simulink model "EMB_LRM"  (R2025a)
settings: Solver=VariableStepAuto  StartTime=0.0  StopTime=10.0  RelTol=1e-3
values from neighbouring files (symbols this model uses):
  cal_u16FailWatchWindow = uint16(20)    [sim_test.m]
  cal_u16FallbackSupportSwapTime = uint16(50)    [sim_test.m]
  cal_u16LaneInitWaitTime = uint16(100)    [sim_test.m]
  cal_u16MasterFallbackSwapThd = uint16(20)    [sim_test.m]
  cal_u16TakeoverTime = uint16(50)    [sim_test.m]
  cal_u8RmtLaneFailThd = uint8(20)    [sim_test.m]
  cal_u8RoleChangeDebounceTime = uint8(10)    [sim_test.m]
settings Model: Creator=wangtianqi  LastModifiedBy=wangtianqi

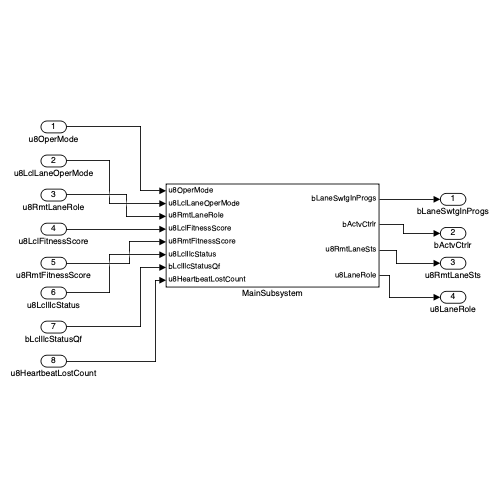
[thumbnail: Simulink's stored preview of the top-level diagram]
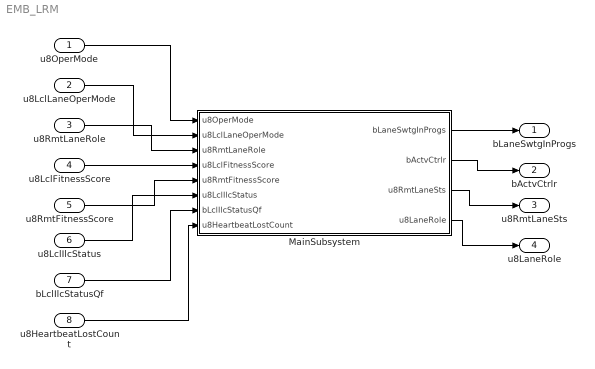
== system EMB_LRM ==
  u8OperMode : Inport  Description=系统运行模式（enum：0 INIT，1 NORMAL_OPERATION，2 LIMP_HOME，3 LIMP_ASIDE，4 CRAWL，5 SHUTTING_DOWN），类型 uint8  OutDataTypeStr=uint8
  u8LclLaneOperMode : Inport  Description=本控制链路运行模式（enum，编码同 OPER MODE），类型 uint8  Port=2  OutDataTypeStr=uint8
  u8RmtLaneRole : Inport  Description=远控制链路当前角色（enum：0 INIT，1 MASTER，2 FALLBACK，3 SUPPORT，4 DISABLED，5 SHUTTING_DOWN），类型 uint8  Port=3  OutDataTypeStr=uint8
  u8LclFitnessScore : Inport  Description=本控制链路健康度得分（62=禁用，255=无效），类型 uint8  Port=4  OutDataTypeStr=uint8
  u8RmtFitnessScore : Inport  Description=远控制链路健康度得分（62=禁用，255=无效），类型 uint8  Port=5  OutDataTypeStr=uint8
  u8LclIlcStatus : Inport  Description=本控制链路 ILC 状态（0x0 Failed，0x1 Normal，0x2 Initialized），类型 uint8  Port=6  OutDataTypeStr=uint8
  bLclIlcStatusQf : Inport  Description=本控制链路状态信号质量（0x0 QF_Full，0x1 QF_Not Full），类型 boolean  Port=7  OutDataTypeStr=boolean
  u8HeartbeatLostCount : Inport  Description=心跳丢失计数（0-255），类型 uint8  Port=8  OutDataTypeStr=uint8
  MainSubsystem : Subsystem  Description=EMB_LRM 主逻辑包装层：SignalAcquisition -> 功能子系统(LRM_MLS / LRM_MLR -> LRM_LSP) -> OutputArbitration -> Out；运行周期 10ms，ASIL-D
  bLaneSwtgInProgs : Outport  Description=控制链路切换进行中标志（0x0 Not Progress，0x1 Progress），类型 boolean  OutDataTypeStr=boolean
  bActvCtrlr : Outport  Description=活动控制器实例标志（0x0 Not Active，0x1 Active），类型 boolean  Port=2  OutDataTypeStr=boolean
  u8RmtLaneSts : Outport  Description=远控制链路状态（0 INITIALISING，1 OPERATING，2 HB_LOST，3 FAILED），类型 uint8  Port=3  OutDataTypeStr=uint8
  u8LaneRole : Outport  Description=本控制链路角色状态（enum：0 UNKNOWN，1 INIT，2 MASTER，3 FALLBACK，4 SUPPORT，5 DISABLED，6 SHUTTING_DOWN），类型 uint8  Port=4  OutDataTypeStr=uint8
  wires:
  MainSubsystem/4(u8LaneRole) -> u8LaneRole/1
  u8RmtLaneRole/1 -> MainSubsystem/3(u8RmtLaneRole)
  u8OperMode/1 -> MainSubsystem/1(u8OperMode)
  MainSubsystem/2(bActvCtrlr) -> bActvCtrlr/1
  MainSubsystem/1(bLaneSwtgInProgs) -> bLaneSwtgInProgs/1
  u8HeartbeatLostCount/1 -> MainSubsystem/8(u8HeartbeatLostCount)
  bLclIlcStatusQf/1 -> MainSubsystem/7(bLclIlcStatusQf)
  u8RmtFitnessScore/1 -> MainSubsystem/5(u8RmtFitnessScore)
  MainSubsystem/3(u8RmtLaneSts) -> u8RmtLaneSts/1
  u8LclFitnessScore/1 -> MainSubsystem/4(u8LclFitnessScore)
  u8LclLaneOperMode/1 -> MainSubsystem/2(u8LclLaneOperMode)
  u8LclIlcStatus/1 -> MainSubsystem/6(u8LclIlcStatus)

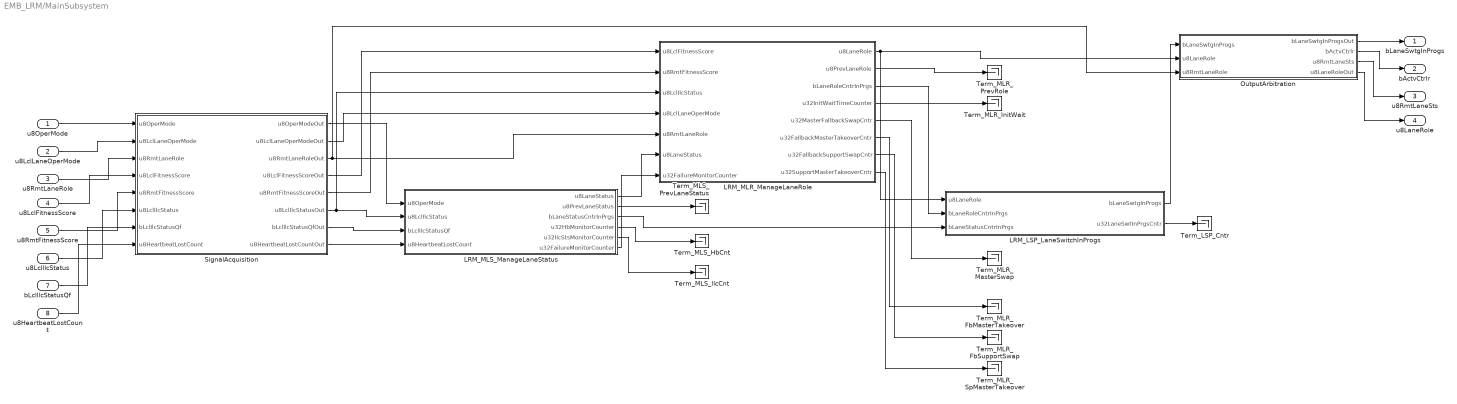
== system EMB_LRM/MainSubsystem ==
  u8OperMode : Inport  OutDataTypeStr=uint8
  u8LclLaneOperMode : Inport  Port=2  OutDataTypeStr=uint8
  u8RmtLaneRole : Inport  Port=3  OutDataTypeStr=uint8
  u8LclFitnessScore : Inport  Port=4  OutDataTypeStr=uint8
  u8RmtFitnessScore : Inport  Port=5  OutDataTypeStr=uint8
  u8LclIlcStatus : Inport  Port=6  OutDataTypeStr=uint8
  bLclIlcStatusQf : Inport  Port=7  OutDataTypeStr=boolean
  u8HeartbeatLostCount : Inport  Port=8  OutDataTypeStr=uint8
  LRM_LSP_LaneSwitchInProgs : Subsystem  Description=检测角色变化并管理切换过渡过程。已实现：LaneRoleChanged=(u8LaneRole != delay)；IfAnyTimerNonZero=bLaneRoleCntrInPrgs OR bLaneStatusCntrInPrgs；切换计数器按优先级 A>B>C：A) 角色变化置计数=1/标志=1；B) 计数>0 时递增，超过 cal_u8RoleChangeDebounceTime 后清零标志并清零计数；C) 任一计数进行中时计数清零、标志=1；否则标志=0。由 Unit Delay / Sum / Relational Operator / Logical Operator / Switch 组合实现
  LRM_MLR_ManageLaneRole : Subsystem  Description=基于健康度得分、ILC 状态、远链路角色与控制链路状态仲裁本链路角色 LaneRole。状态机采用 boolean 门控 Stateflow 模式：全部比较/计数/条件组合在 Simulink 内完成（Relational Operator、Unit Delay+Sum+Switch 计数器、Logical Operator），Chart(MLR_STM) 仅接收 boolean 条件（bOperShutdown/bLclDisabled/bExitInitMaster/bFbToMasterImm 等 26 路）并执行 6 状态（INIT/MASTER/FALLBACK/SUPPORT/DISABLED/SHUTTING_DOWN）转移，输出 u8LaneRole 状态编码；prevLaneRole、LaneRoleCntrInPrgs、各切换/接管计数器在 Simulink 由状态输出派生
  LRM_MLS_ManageLaneStatus : Subsystem  Description=监控 LCL ILC STATUS_QF、OPER MODE 与 LCL ILC STATUS，判定控制链路健康状态 LaneStatus。已实现：MLR_HB_Failure=(HEARTBEAT LOST COUNT != delay+1 mod 256)；计数器 HbMonitorCounter/ILCStsMonitorCounter/FailureMonitorCounter 仅监控激活时计数（Hb/Failure 以 HB_Failure>0 增量，ILC 以 QF!=FULL 增量）；四状态机 INIT/Operating/HbLost/Failed（优先级 Operating>Failed>HbLost）：INIT 在 OPER MODE 为 NORMAL/LIMP_HOME/LIMP_ASIDE/CRAWL 时激活监控；Operating 需 QF_FULL 且 HB_Failure=0；Failed 需 abs(int32(Hb-ILC))<=5 且 FailureCnt>=cal_u8RmtLaneFailThd；HbLost 需 HbCnt>=cal_u8RmtLaneFailThd 且 FailureCnt>=cal_u8RmtLaneFailThd（或从 Failed 且 QF_FULL）；进入非 Operating 状态清零计数器；LaneStatusCntrInPrgs=HB_Failure>0 OR QF!=FULL。由 Unit Delay / Sum / Relational Operator / Logical Operator / Switch 组合实现
  OutputArbitration : Subsystem  Description=输出仲裁与合并：bLaneSwtgInProgs 由 LSP 直通；bActvCtrlr=(u8LaneRole==LN_ROLE_MASTER)（Relational Operator 判等）；u8RmtLaneSts 暂由 u8RmtLaneRole 直通占位（映射待确认）；u8LaneRole 直通
  SignalAcquisition : Subsystem  Description=信号调理与类型转换：本期 8 路输入类型已与内部约定一致，按原类型直通；后续类型不一致时在此集中加入 Data Type Conversion
  Term_LSP_Cntr : Terminator
  Term_MLR_FbMasterTakeover : Terminator
  Term_MLR_FbSupportSwap : Terminator
  Term_MLR_InitWait : Terminator
  Term_MLR_MasterSwap : Terminator
  Term_MLR_PrevRole : Terminator
  Term_MLR_SpMasterTakeover : Terminator
  Term_MLS_HbCnt : Terminator
  Term_MLS_IlcCnt : Terminator
  Term_MLS_PrevLaneStatus : Terminator
  bLaneSwtgInProgs : Outport  OutDataTypeStr=boolean
  bActvCtrlr : Outport  Port=2  OutDataTypeStr=boolean
  u8RmtLaneSts : Outport  Port=3  OutDataTypeStr=uint8
  u8LaneRole : Outport  Port=4  OutDataTypeStr=uint8
  wires:
  LRM_LSP_LaneSwitchInProgs/2(u32LaneSwtInPrgsCntr) -> Term_LSP_Cntr/1
  LRM_MLR_ManageLaneRole/4(u32InitWaitTimeCounter) -> Term_MLR_InitWait/1
  LRM_MLR_ManageLaneRole/3(bLaneRoleCntrInPrgs) -> LRM_LSP_LaneSwitchInProgs/2(bLaneRoleCntrInPrgs)
  OutputArbitration/3(u8RmtLaneSts) -> u8RmtLaneSts/1
  LRM_MLR_ManageLaneRole/2(u8PrevLaneRole) -> Term_MLR_PrevRole/1
  LRM_MLS_ManageLaneStatus/6(u32FailureMonitorCounter) -> LRM_MLR_ManageLaneRole/7(u32FailureMonitorCounter)
  LRM_LSP_LaneSwitchInProgs/1(bLaneSwtgInProgs) -> OutputArbitration/1(bLaneSwtgInProgs)
  u8OperMode/1 -> SignalAcquisition/1(u8OperMode)
  LRM_MLS_ManageLaneStatus/5(u32IlcStsMonitorCounter) -> Term_MLS_IlcCnt/1
  LRM_MLR_ManageLaneRole/7(u32FallbackSupportSwapCntr) -> Term_MLR_FbSupportSwap/1
  LRM_MLS_ManageLaneStatus/4(u32HbMonitorCounter) -> Term_MLS_HbCnt/1
  OutputArbitration/2(bActvCtrlr) -> bActvCtrlr/1
  LRM_MLS_ManageLaneStatus/2(u8PrevLaneStatus) -> Term_MLS_PrevLaneStatus/1
  OutputArbitration/1(bLaneSwtgInProgsOut) -> bLaneSwtgInProgs/1
  bLclIlcStatusQf/1 -> SignalAcquisition/7(bLclIlcStatusQf)
  SignalAcquisition/8(u8HeartbeatLostCountOut) -> LRM_MLS_ManageLaneStatus/4(u8HeartbeatLostCount)
  LRM_MLR_ManageLaneRole/8(u32SupportMasterTakeoverCntr) -> Term_MLR_SpMasterTakeover/1
  LRM_MLR_ManageLaneRole/1(u8LaneRole) -> LRM_LSP_LaneSwitchInProgs/1(u8LaneRole), OutputArbitration/2(u8LaneRole)
  u8RmtFitnessScore/1 -> SignalAcquisition/5(u8RmtFitnessScore)
  SignalAcquisition/4(u8LclFitnessScoreOut) -> LRM_MLR_ManageLaneRole/1(u8LclFitnessScore)
  SignalAcquisition/3(u8RmtLaneRoleOut) -> OutputArbitration/3(u8RmtLaneRole), LRM_MLR_ManageLaneRole/5(u8RmtLaneRole)
  SignalAcquisition/2(u8LclLaneOperModeOut) -> LRM_MLR_ManageLaneRole/4(u8LclLaneOperMode)
  LRM_MLS_ManageLaneStatus/1(u8LaneStatus) -> LRM_MLR_ManageLaneRole/6(u8LaneStatus)
  SignalAcquisition/7(bLclIlcStatusQfOut) -> LRM_MLS_ManageLaneStatus/3(bLclIlcStatusQf)
  u8HeartbeatLostCount/1 -> SignalAcquisition/8(u8HeartbeatLostCount)
  SignalAcquisition/1(u8OperModeOut) -> LRM_MLS_ManageLaneStatus/1(u8OperMode)
  SignalAcquisition/5(u8RmtFitnessScoreOut) -> LRM_MLR_ManageLaneRole/2(u8RmtFitnessScore)
  u8LclIlcStatus/1 -> SignalAcquisition/6(u8LclIlcStatus)
  LRM_MLR_ManageLaneRole/5(u32MasterFallbackSwapCntr) -> Term_MLR_MasterSwap/1
  SignalAcquisition/6(u8LclIlcStatusOut) -> LRM_MLS_ManageLaneStatus/2(u8LclIlcStatus), LRM_MLR_ManageLaneRole/3(u8LclIlcStatus)
  u8LclFitnessScore/1 -> SignalAcquisition/4(u8LclFitnessScore)
  OutputArbitration/4(u8LaneRoleOut) -> u8LaneRole/1
  u8RmtLaneRole/1 -> SignalAcquisition/3(u8RmtLaneRole)
  LRM_MLS_ManageLaneStatus/3(bLaneStatusCntrInPrgs) -> LRM_LSP_LaneSwitchInProgs/3(bLaneStatusCntrInPrgs)
  LRM_MLR_ManageLaneRole/6(u32FallbackMasterTakeoverCntr) -> Term_MLR_FbMasterTakeover/1
  u8LclLaneOperMode/1 -> SignalAcquisition/2(u8LclLaneOperMode)

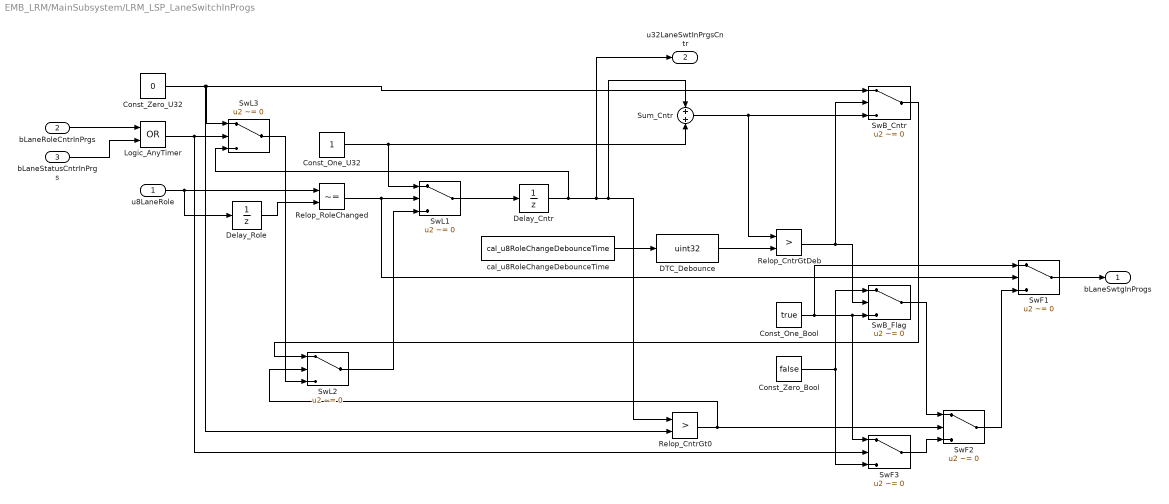
== system EMB_LRM/MainSubsystem/LRM_LSP_LaneSwitchInProgs ==
  u8LaneRole : Inport
  bLaneRoleCntrInPrgs : Inport  Port=2
  bLaneStatusCntrInPrgs : Inport  Port=3
  Const_One_Bool : Constant  Value=true  OutDataTypeStr=boolean
  Const_One_U32 : Constant  OutDataTypeStr=uint32
  Const_Zero_Bool : Constant  Value=false  OutDataTypeStr=boolean
  Const_Zero_U32 : Constant  Value=0  OutDataTypeStr=uint32
  DTC_Debounce : DataTypeConversion  OutDataTypeStr=uint32  SaturateOnIntegerOverflow=off  RndMeth=Floor
  Delay_Cntr : UnitDelay  SampleTime=0.01  HasFrameUpgradeWarning=on
  Delay_Role : UnitDelay  SampleTime=0.01  HasFrameUpgradeWarning=on
  Logic_AnyTimer : Logic  Operator=OR  AllPortsSameDT=off  OutDataTypeStr=boolean
  Relop_CntrGt0 : RelationalOperator  Operator=>  OutDataTypeStr=boolean  RndMeth=Simplest  InputSameDT=off
  Relop_CntrGtDeb : RelationalOperator  Operator=>  OutDataTypeStr=boolean  RndMeth=Simplest  InputSameDT=off
  Relop_RoleChanged : RelationalOperator  Operator=~=  OutDataTypeStr=boolean  RndMeth=Simplest  InputSameDT=off
  Sum_Cntr : Sum  OutDataTypeStr=uint32
  SwB_Cntr : Switch  Criteria=u2 ~= 0  OutDataTypeStr=uint32  SaturateOnIntegerOverflow=off  InputSameDT=off
  SwB_Flag : Switch  Criteria=u2 ~= 0  OutDataTypeStr=boolean  SaturateOnIntegerOverflow=off  InputSameDT=off
  SwF1 : Switch  Criteria=u2 ~= 0  OutDataTypeStr=boolean  SaturateOnIntegerOverflow=off  InputSameDT=off
  SwF2 : Switch  Criteria=u2 ~= 0  OutDataTypeStr=boolean  SaturateOnIntegerOverflow=off  InputSameDT=off
  SwF3 : Switch  Criteria=u2 ~= 0  OutDataTypeStr=boolean  SaturateOnIntegerOverflow=off  InputSameDT=off
  SwL1 : Switch  Criteria=u2 ~= 0  OutDataTypeStr=uint32  SaturateOnIntegerOverflow=off  InputSameDT=off
  SwL2 : Switch  Criteria=u2 ~= 0  OutDataTypeStr=uint32  SaturateOnIntegerOverflow=off  InputSameDT=off
  SwL3 : Switch  Criteria=u2 ~= 0  OutDataTypeStr=uint32  SaturateOnIntegerOverflow=off  InputSameDT=off
  cal_u8RoleChangeDebounceTime : Constant  Description=cal_u8RoleChangeDebounceTime；角色切换防抖时间阈值（周期数），对应 ROLE_CHANGE_DEBOUNCE_TIME；uint8；cycle；0..255；默认 10  Value=cal_u8RoleChangeDebounceTime  OutDataTypeStr=uint8
  bLaneSwtgInProgs : Outport
  u32LaneSwtInPrgsCntr : Outport  Port=2
  wires:
  SwF1/1 -> bLaneSwtgInProgs/1
  SwF2/1 -> SwF1/3
  SwF3/1 -> SwF2/3
  Const_Zero_Bool/1 -> SwB_Flag/1, SwF3/3
  Relop_CntrGtDeb/1 -> SwB_Cntr/2, SwB_Flag/2
  DTC_Debounce/1 -> Relop_CntrGtDeb/2
  Sum_Cntr/1 -> Relop_CntrGtDeb/1, SwB_Cntr/3
  u8LaneRole/1 -> Delay_Role/1, Relop_RoleChanged/1
  cal_u8RoleChangeDebounceTime/1 -> DTC_Debounce/1
  SwL2/1 -> SwL1/3
  Logic_AnyTimer/1 -> SwL3/2, SwF3/2
  Delay_Cntr/1 -> Sum_Cntr/1, Relop_CntrGt0/1, u32LaneSwtInPrgsCntr/1, SwL3/3
  Relop_RoleChanged/1 -> SwL1/2, SwF1/2
  SwL1/1 -> Delay_Cntr/1
  SwB_Flag/1 -> SwF2/1
  Const_One_U32/1 -> SwL1/1, Sum_Cntr/2
  Delay_Role/1 -> Relop_RoleChanged/2
  SwB_Cntr/1 -> SwL2/1
  Relop_CntrGt0/1 -> SwF2/2, SwL2/2
  bLaneStatusCntrInPrgs/1 -> Logic_AnyTimer/2
  Const_Zero_U32/1 -> SwL3/1, SwB_Cntr/1, Relop_CntrGt0/2
  SwL3/1 -> SwL2/3
  Const_One_Bool/1 -> SwB_Flag/3, SwF3/1, SwF1/1
  bLaneRoleCntrInPrgs/1 -> Logic_AnyTimer/1

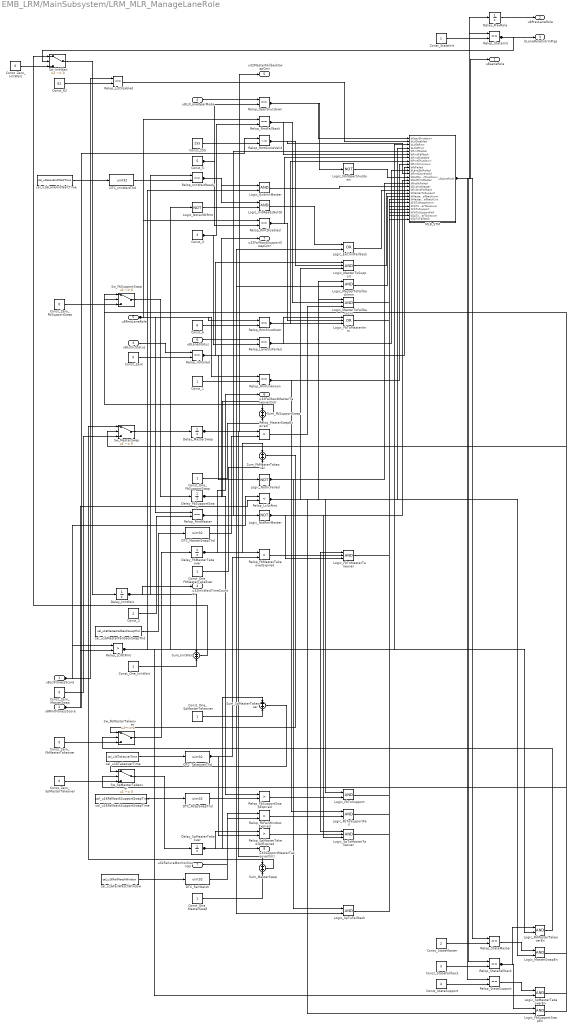
== system EMB_LRM/MainSubsystem/LRM_MLR_ManageLaneRole ==
  u8LclFitnessScore : Inport  OutDataTypeStr=uint8
  u8RmtFitnessScore : Inport  Port=2  OutDataTypeStr=uint8
  u8LclIlcStatus : Inport  Port=3  OutDataTypeStr=uint8
  u8LclLaneOperMode : Inport  Port=4  OutDataTypeStr=uint8
  u8RmtLaneRole : Inport  Port=5  OutDataTypeStr=uint8
  u8LaneStatus : Inport  Port=6  OutDataTypeStr=uint8
  u32FailureMonitorCounter : Inport  Port=7  OutDataTypeStr=uint32
  Const_1 : Constant  OutDataTypeStr=uint8
  Const_2 : Constant  Value=2  OutDataTypeStr=uint8
  Const_255 : Constant  Value=255  OutDataTypeStr=uint8
  Const_3 : Constant  Value=3  OutDataTypeStr=uint8
  Const_5 : Constant  Value=5  OutDataTypeStr=uint8
  Const_6 : Constant  Value=6  OutDataTypeStr=uint8
  Const_62 : Constant  Value=62  OutDataTypeStr=uint8
  Const_One_FbMasterTakeover : Constant  OutDataTypeStr=uint32
  Const_One_FbSupportSwap : Constant  OutDataTypeStr=uint32
  Const_One_InitWait : Constant  OutDataTypeStr=uint32
  Const_One_MasterSwap : Constant  OutDataTypeStr=uint32
  Const_One_SpMasterTakeover : Constant  OutDataTypeStr=uint32
  Const_StateFallback : Constant  Value=3  OutDataTypeStr=uint8
  Const_StateInit : Constant  OutDataTypeStr=uint8
  Const_StateMaster : Constant  Value=2  OutDataTypeStr=uint8
  Const_StateSupport : Constant  Value=4  OutDataTypeStr=uint8
  Const_Zero : Constant  Value=0  OutDataTypeStr=uint8
  Const_Zero_FbMasterTakeover : Constant  Value=0  OutDataTypeStr=uint32
  Const_Zero_FbSupportSwap : Constant  Value=0  OutDataTypeStr=uint32
  Const_Zero_InitWait : Constant  Value=0  OutDataTypeStr=uint32
  Const_Zero_MasterSwap : Constant  Value=0  OutDataTypeStr=uint32
  Const_Zero_SpMasterTakeover : Constant  Value=0  OutDataTypeStr=uint32
  DTC_FailWatch : DataTypeConversion  OutDataTypeStr=uint32  SaturateOnIntegerOverflow=off  RndMeth=Floor
  DTC_FbSpSwapThd : DataTypeConversion  OutDataTypeStr=uint32  SaturateOnIntegerOverflow=off  RndMeth=Floor
  DTC_InitWaitThd : DataTypeConversion  OutDataTypeStr=uint32  SaturateOnIntegerOverflow=off  RndMeth=Floor
  DTC_MasterSwapThd : DataTypeConversion  OutDataTypeStr=uint32  SaturateOnIntegerOverflow=off  RndMeth=Floor
  DTC_TakeoverThd : DataTypeConversion  OutDataTypeStr=uint32  SaturateOnIntegerOverflow=off  RndMeth=Floor
  Delay_FbMasterTakeover : UnitDelay  SampleTime=0.01  HasFrameUpgradeWarning=on
  Delay_FbSupportSwap : UnitDelay  SampleTime=0.01  HasFrameUpgradeWarning=on
  Delay_InitWait : UnitDelay  SampleTime=0.01  HasFrameUpgradeWarning=on
  Delay_MasterSwap : UnitDelay  SampleTime=0.01  HasFrameUpgradeWarning=on
  Delay_PrevRole : UnitDelay  InitialCondition=1  SampleTime=0.01  HasFrameUpgradeWarning=on
  Delay_SpMasterTakeover : UnitDelay  SampleTime=0.01  HasFrameUpgradeWarning=on
  Logic_ExitInitFallback : Logic  Operator=OR  AllPortsSameDT=off  OutDataTypeStr=boolean
  Logic_ExitInitMaster : Logic  AllPortsSameDT=off  OutDataTypeStr=boolean
  Logic_FbMasterTakeoverEn : Logic  AllPortsSameDT=off  OutDataTypeStr=boolean
  Logic_FbSupportSwapEn : Logic  AllPortsSameDT=off  OutDataTypeStr=boolean
  Logic_FbToMasterImm : Logic  Operator=OR  Inputs=3  AllPortsSameDT=off  OutDataTypeStr=boolean
  Logic_FbToMasterTakeover : Logic  Inputs=3  AllPortsSameDT=off  OutDataTypeStr=boolean
  Logic_FbToSupport : Logic  AllPortsSameDT=off  OutDataTypeStr=boolean
  Logic_FbToSupportFail : Logic  AllPortsSameDT=off  OutDataTypeStr=boolean
  Logic_InitReadyNotGt : Logic  AllPortsSameDT=off  OutDataTypeStr=boolean
  Logic_MasterSwapEn : Logic  AllPortsSameDT=off  OutDataTypeStr=boolean
  Logic_MasterToFallbackCnt : Logic  Inputs=3  AllPortsSameDT=off  OutDataTypeStr=boolean
  Logic_MasterToFallbackImm : Logic  AllPortsSameDT=off  OutDataTypeStr=boolean
  Logic_MasterToSupport : Logic  Inputs=3  AllPortsSameDT=off  OutDataTypeStr=boolean
  Logic_NotIlcFailed : Logic  Operator=NOT  Inputs=1  AllPortsSameDT=off  OutDataTypeStr=boolean
  Logic_NotLclGtRmt : Logic  Operator=NOT  Inputs=1  AllPortsSameDT=off  OutDataTypeStr=boolean
  Logic_NotOperShutdown : Logic  Operator=NOT  Inputs=1  AllPortsSameDT=off  OutDataTypeStr=boolean
  Logic_NotRmtMaster : Logic  Operator=NOT  Inputs=1  AllPortsSameDT=off  OutDataTypeStr=boolean
  Logic_SpMasterTakeoverEn : Logic  AllPortsSameDT=off  OutDataTypeStr=boolean
  Logic_SpToFallback : Logic  AllPortsSameDT=off  OutDataTypeStr=boolean
  Logic_SpToMasterTakeover : Logic  Inputs=3  AllPortsSameDT=off  OutDataTypeStr=boolean
  MLR_STM : Stateflow chart  Description=MLR 角色仲裁状态机（boolean 门控 Stateflow）：26 路 boolean 条件输入，6 状态（INIT/MASTER/FALLBACK/SUPPORT/DISABLED/SHUTTING_DOWN）转移，输出 u8LaneRole 状态编码；全部逻辑判断在 Simulink 侧完成  TreatAsAtomicUnit=on
  Relop_FbFailWindowExpired : RelationalOperator  Operator=>  OutDataTypeStr=boolean  RndMeth=Simplest  InputSameDT=off
  Relop_FbMasterTakeoverExpired : RelationalOperator  Operator=>  OutDataTypeStr=boolean  RndMeth=Simplest  InputSameDT=off
  Relop_FbSupportSwapExpired : RelationalOperator  Operator=>  OutDataTypeStr=boolean  RndMeth=Simplest  InputSameDT=off
  Relop_IlcFailed : RelationalOperator  Operator===  OutDataTypeStr=boolean  RndMeth=Simplest  InputSameDT=off
  Relop_InitWaitReady : RelationalOperator  OutDataTypeStr=boolean  RndMeth=Simplest  InputSameDT=off
  Relop_LaneStsFailed : RelationalOperator  Operator===  OutDataTypeStr=boolean  RndMeth=Simplest  InputSameDT=off
  Relop_LclDisabled : RelationalOperator  Operator===  OutDataTypeStr=boolean  RndMeth=Simplest  InputSameDT=off
  Relop_LclGtRmt : RelationalOperator  Operator=>  OutDataTypeStr=boolean  RndMeth=Simplest  InputSameDT=off
  Relop_LclLtRmt : RelationalOperator  Operator=<  OutDataTypeStr=boolean  RndMeth=Simplest  InputSameDT=off
  Relop_MasterSwapExpired : RelationalOperator  Operator=>  OutDataTypeStr=boolean  RndMeth=Simplest  InputSameDT=off
  Relop_OperShutdown : RelationalOperator  Operator===  OutDataTypeStr=boolean  RndMeth=Simplest  InputSameDT=off
  Relop_RmtDisabled : RelationalOperator  Operator===  OutDataTypeStr=boolean  RndMeth=Simplest  InputSameDT=off
  Relop_RmtFallback : RelationalOperator  Operator===  OutDataTypeStr=boolean  RndMeth=Simplest  InputSameDT=off
  Relop_RmtMaster : RelationalOperator  Operator===  OutDataTypeStr=boolean  RndMeth=Simplest  InputSameDT=off
  Relop_RmtScoreValid : RelationalOperator  Operator=~=  OutDataTypeStr=boolean  RndMeth=Simplest  InputSameDT=off
  Relop_RmtShutdown : RelationalOperator  Operator===  OutDataTypeStr=boolean  RndMeth=Simplest  InputSameDT=off
  Relop_RmtUnknown : RelationalOperator  Operator===  OutDataTypeStr=boolean  RndMeth=Simplest  InputSameDT=off
  Relop_SpMasterTakeoverExpired : RelationalOperator  Operator=>  OutDataTypeStr=boolean  RndMeth=Simplest  InputSameDT=off
  Relop_StateFallback : RelationalOperator  Operator===  OutDataTypeStr=boolean  RndMeth=Simplest  InputSameDT=off
  Relop_StateInit : RelationalOperator  Operator===  OutDataTypeStr=boolean  RndMeth=Simplest  InputSameDT=off
  Relop_StateMaster : RelationalOperator  Operator===  OutDataTypeStr=boolean  RndMeth=Simplest  InputSameDT=off
  Relop_StateSupport : RelationalOperator  Operator===  OutDataTypeStr=boolean  RndMeth=Simplest  InputSameDT=off
  Sum_FbMasterTakeover : Sum  OutDataTypeStr=uint32
  Sum_FbSupportSwap : Sum  OutDataTypeStr=uint32
  Sum_InitWait : Sum  OutDataTypeStr=uint32
  Sum_MasterSwap : Sum  OutDataTypeStr=uint32
  Sum_SpMasterTakeover : Sum  OutDataTypeStr=uint32
  Sw_FbMasterTakeover : Switch  Criteria=u2 ~= 0  OutDataTypeStr=uint32  SaturateOnIntegerOverflow=off  InputSameDT=off
  Sw_FbSupportSwap : Switch  Criteria=u2 ~= 0  OutDataTypeStr=uint32  SaturateOnIntegerOverflow=off  InputSameDT=off
  Sw_InitWait : Switch  Criteria=u2 ~= 0  OutDataTypeStr=uint32  SaturateOnIntegerOverflow=off  InputSameDT=off
  Sw_MasterSwap : Switch  Criteria=u2 ~= 0  OutDataTypeStr=uint32  SaturateOnIntegerOverflow=off  InputSameDT=off
  Sw_SpMasterTakeover : Switch  Criteria=u2 ~= 0  OutDataTypeStr=uint32  SaturateOnIntegerOverflow=off  InputSameDT=off
  cal_u16FailWatchWindow : Constant  Description=cal_u16FailWatchWindow；故障监控窗口阈值，对应 FAIL_WATCH_WINDOW；uint16；cycle；默认 20（待确认）  Value=cal_u16FailWatchWindow  OutDataTypeStr=uint16
  cal_u16FallbackSupportSwapTime : Constant  Description=cal_u16FallbackSupportSwapTime；Fallback 向 Support 降级时间阈值，对应 LANE_FALLBACK_SUPPORT_SWAP_TIME；uint16；cycle；默认 50（待确认）  Value=cal_u16FallbackSupportSwapTime  OutDataTypeStr=uint16
  cal_u16LaneInitWaitTime : Constant  Description=cal_u16LaneInitWaitTime；初始化等待时间阈值（周期数），对应 LANE_INIT_WAIT_TIME；uint16；cycle；默认 100（待确认）  Value=cal_u16LaneInitWaitTime  OutDataTypeStr=uint16
  cal_u16MasterFallbackSwapThd : Constant  Description=cal_u16MasterFallbackSwapThd；Master 向 Fallback 切换计数阈值；uint16；cycle；默认 20  Value=cal_u16MasterFallbackSwapThd  OutDataTypeStr=uint16
  cal_u16TakeoverTime : Constant  Description=cal_u16TakeoverTime；接管时间阈值（周期数），对应 TAKEOVER_TIME；uint16；cycle；默认 50（待确认）  Value=cal_u16TakeoverTime  OutDataTypeStr=uint16
  u8LaneRole : Outport  OutDataTypeStr=uint8
  u8PrevLaneRole : Outport  Port=2  OutDataTypeStr=uint8
  bLaneRoleCntrInPrgs : Outport  Port=3  OutDataTypeStr=boolean
  u32InitWaitTimeCounter : Outport  Port=4  OutDataTypeStr=uint32
  u32MasterFallbackSwapCntr : Outport  Port=5  OutDataTypeStr=uint32
  u32FallbackMasterTakeoverCntr : Outport  Port=6  OutDataTypeStr=uint32
  u32FallbackSupportSwapCntr : Outport  Port=7  OutDataTypeStr=uint32
  u32SupportMasterTakeoverCntr : Outport  Port=8  OutDataTypeStr=uint32
  wires:
  DTC_InitWaitThd/1 -> Relop_InitWaitReady/2
  Relop_SpMasterTakeoverExpired/1 -> Logic_SpToMasterTakeover/2
  Logic_FbToMasterImm/1 -> MLR_STM/21(bFbToMasterImm)
  Const_2/1 -> Relop_RmtMaster/2
  Logic_FbToSupport/1 -> MLR_STM/23(bFbToSupport)
  u8LaneStatus/1 -> Relop_LaneStsFailed/1
  Const_255/1 -> Relop_RmtScoreValid/2
  Const_6/1 -> Relop_RmtShutdown/2
  Logic_MasterToFallbackImm/1 -> MLR_STM/19(bMasterToFallbackImm)
  Sum_FbMasterTakeover/1 -> Sw_FbMasterTakeover/1
  Const_62/1 -> Relop_LclDisabled/2
  Logic_FbToSupportFail/1 -> MLR_STM/24(bFbToSupportFail)
  Relop_StateSupport/1 -> Logic_SpMasterTakeoverEn/1
  Sum_MasterSwap/1 -> Sw_MasterSwap/1
  Sw_SpMasterTakeover/1 -> Delay_SpMasterTakeover/1
  Const_Zero_MasterSwap/1 -> Sw_MasterSwap/3
  Const_1/1 -> Relop_RmtUnknown/2
  DTC_FbSpSwapThd/1 -> Relop_FbSupportSwapExpired/2
  cal_u16MasterFallbackSwapThd/1 -> DTC_MasterSwapThd/1
  Relop_OperShutdown/1 -> Logic_NotOperShutdown/1, MLR_STM/1(bOperShutdown)
  Logic_SpToFallback/1 -> MLR_STM/26(bSpToFallback)
  DTC_MasterSwapThd/1 -> Relop_MasterSwapExpired/2
  Logic_MasterToFallbackCnt/1 -> MLR_STM/20(bMasterToFallbackCnt)
  Const_StateFallback/1 -> Relop_StateFallback/2
  Relop_StateMaster/1 -> Logic_MasterSwapEn/1
  Const_Zero_FbSupportSwap/1 -> Sw_FbSupportSwap/3
  Const_StateSupport/1 -> Relop_StateSupport/2
  Sw_InitWait/1 -> Delay_InitWait/1
  Const_StateMaster/1 -> Relop_StateMaster/2
  Logic_NotLclGtRmt/1 -> Logic_InitReadyNotGt/2
  Sw_MasterSwap/1 -> Delay_MasterSwap/1
  Logic_MasterToSupport/1 -> MLR_STM/18(bMasterToSupport)
  DTC_FailWatch/1 -> Relop_FbFailWindowExpired/2
  Delay_PrevRole/1 -> u8PrevLaneRole/1
  u32FailureMonitorCounter/1 -> Relop_FbFailWindowExpired/1
  Sw_FbSupportSwap/1 -> Delay_FbSupportSwap/1
  Sum_FbSupportSwap/1 -> Sw_FbSupportSwap/1
  DTC_TakeoverThd/1 -> Relop_SpMasterTakeoverExpired/2, Relop_FbMasterTakeoverExpired/2
  Relop_FbMasterTakeoverExpired/1 -> Logic_FbToMasterTakeover/2
  Const_5/1 -> Relop_RmtDisabled/2, Relop_OperShutdown/2
  Const_One_InitWait/1 -> Sum_InitWait/2
  Relop_LclDisabled/1 -> MLR_STM/2(bLclDisabled)
  Const_Zero_InitWait/1 -> Sw_InitWait/3
  Logic_NotIlcFailed/1 -> MLR_STM/15(bNotIlcFailed), Logic_SpToFallback/1
  Relop_LaneStsFailed/1 -> Logic_FbToMasterImm/1, MLR_STM/11(bLaneStsFailed)
  Const_Zero_FbMasterTakeover/1 -> Sw_FbMasterTakeover/3
  u8LclIlcStatus/1 -> Relop_IlcFailed/1
  cal_u16TakeoverTime/1 -> DTC_TakeoverThd/1
  Logic_NotOperShutdown/1 -> MLR_STM/13(bNotOperShutdown)
  Const_One_FbMasterTakeover/1 -> Sum_FbMasterTakeover/2
  Const_3/1 -> Relop_RmtFallback/2, Relop_LaneStsFailed/2
  Relop_InitWaitReady/1 -> Logic_InitReadyNotGt/1, Logic_ExitInitMaster/1
  Const_Zero_SpMasterTakeover/1 -> Sw_SpMasterTakeover/3
  cal_u16FailWatchWindow/1 -> DTC_FailWatch/1
  u8LclFitnessScore/1 -> Relop_LclDisabled/1, Relop_LclGtRmt/1, Relop_LclLtRmt/1
  Relop_StateFallback/1 -> Logic_FbSupportSwapEn/1, Logic_FbMasterTakeoverEn/1
  Relop_MasterSwapExpired/1 -> Logic_MasterToFallbackCnt/3
  Logic_NotRmtMaster/1 -> Logic_SpToMasterTakeover/3, Logic_FbToMasterTakeover/3, MLR_STM/14(bNotRmtMaster)
  cal_u16LaneInitWaitTime/1 -> DTC_InitWaitThd/1
  u8RmtFitnessScore/1 -> Relop_LclGtRmt/2, Relop_LclLtRmt/2, Relop_RmtScoreValid/1
  u8RmtLaneRole/1 -> Relop_RmtUnknown/1, Relop_RmtMaster/1, Relop_RmtShutdown/1, Relop_RmtFallback/1, Relop_RmtDisabled/1
  u8LclLaneOperMode/1 -> Relop_OperShutdown/1
  Delay_FbMasterTakeover/1 -> u32FallbackMasterTakeoverCntr/1, Relop_FbMasterTakeoverExpired/1, Sum_FbMasterTakeover/1
  Logic_FbMasterTakeoverEn/1 -> Sw_FbMasterTakeover/2
  Relop_StateInit/1 -> bLaneRoleCntrInPrgs/1, Sw_InitWait/2
  MLR_STM/1(u8LaneRole) -> Relop_StateFallback/1, Relop_StateMaster/1, Delay_PrevRole/1, Relop_StateSupport/1, Relop_StateInit/1, u8LaneRole/1
  Relop_LclLtRmt/1 -> Logic_MasterToFallbackCnt/1, Logic_MasterToSupport/3, Logic_FbToSupport/1, Logic_MasterToFallbackImm/1, Logic_FbSupportSwapEn/2, Logic_MasterSwapEn/2, MLR_STM/4(bLclLtRmt)
  Relop_RmtFallback/1 -> Logic_MasterToFallbackCnt/2, MLR_STM/6(bRmtFallback)
  Relop_LclGtRmt/1 -> Logic_NotLclGtRmt/1, Logic_SpToMasterTakeover/1, Logic_FbToMasterTakeover/1, MLR_STM/3(bLclGtRmt), Logic_SpMasterTakeoverEn/2, Logic_ExitInitMaster/2, Logic_FbMasterTakeoverEn/2
  Relop_FbSupportSwapExpired/1 -> Logic_FbToSupport/2
  Const_One_SpMasterTakeover/1 -> Sum_SpMasterTakeover/2
  Delay_MasterSwap/1 -> Relop_MasterSwapExpired/1, u32MasterFallbackSwapCntr/1, Sum_MasterSwap/1
  Logic_SpToMasterTakeover/1 -> MLR_STM/25(bSpToMasterTakeover)
  Relop_RmtDisabled/1 -> Logic_FbToMasterImm/2, MLR_STM/7(bRmtDisabled)
  Logic_MasterSwapEn/1 -> Sw_MasterSwap/2
  Sw_FbMasterTakeover/1 -> Delay_FbMasterTakeover/1
  Const_One_MasterSwap/1 -> Sum_MasterSwap/2
  Relop_RmtMaster/1 -> Logic_MasterToFallbackImm/2, Logic_NotRmtMaster/1, Logic_ExitInitFallback/2, MLR_STM/5(bRmtMaster), Logic_SpToFallback/2
  Delay_InitWait/1 -> u32InitWaitTimeCounter/1, Relop_InitWaitReady/1, Sum_InitWait/1
  Relop_RmtShutdown/1 -> Logic_FbToMasterImm/3, MLR_STM/8(bRmtShutdown)
  Logic_ExitInitMaster/1 -> MLR_STM/16(bExitInitMaster)
  Relop_FbFailWindowExpired/1 -> Logic_FbToSupportFail/2
  Logic_InitReadyNotGt/1 -> Logic_ExitInitFallback/1
  Const_One_FbSupportSwap/1 -> Sum_FbSupportSwap/2
  Delay_FbSupportSwap/1 -> u32FallbackSupportSwapCntr/1, Relop_FbSupportSwapExpired/1, Sum_FbSupportSwap/1
  Delay_SpMasterTakeover/1 -> Relop_SpMasterTakeoverExpired/1, u32SupportMasterTakeoverCntr/1, Sum_SpMasterTakeover/1
  Const_Zero/1 -> Relop_IlcFailed/2
  Logic_ExitInitFallback/1 -> MLR_STM/17(bExitInitFallback)
  Relop_RmtScoreValid/1 -> Logic_MasterToSupport/2, MLR_STM/12(bRmtScoreValid)
  Sum_InitWait/1 -> Sw_InitWait/1
  Const_StateInit/1 -> Relop_StateInit/2
  Relop_IlcFailed/1 -> Logic_NotIlcFailed/1, MLR_STM/10(bIlcFailed), Logic_MasterToSupport/1
  Relop_RmtUnknown/1 -> Logic_FbToSupportFail/1, MLR_STM/9(bRmtUnknown)
  Sum_SpMasterTakeover/1 -> Sw_SpMasterTakeover/1
  Logic_FbSupportSwapEn/1 -> Sw_FbSupportSwap/2
  Logic_FbToMasterTakeover/1 -> MLR_STM/22(bFbToMasterTakeover)
  cal_u16FallbackSupportSwapTime/1 -> DTC_FbSpSwapThd/1
  Logic_SpMasterTakeoverEn/1 -> Sw_SpMasterTakeover/2

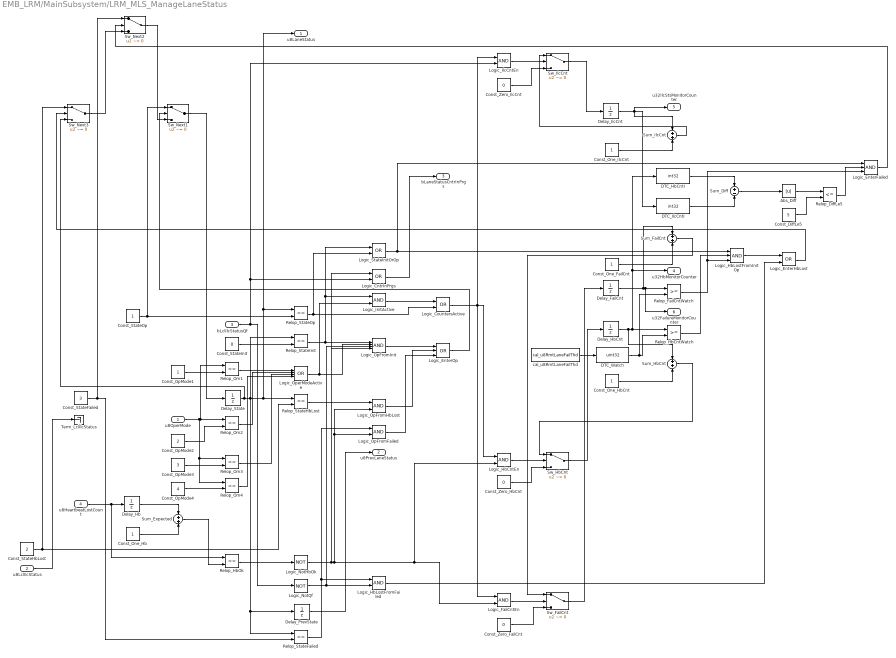
== system EMB_LRM/MainSubsystem/LRM_MLS_ManageLaneStatus ==
  u8OperMode : Inport
  u8LclIlcStatus : Inport  Port=2
  bLclIlcStatusQf : Inport  Port=3
  u8HeartbeatLostCount : Inport  Port=4
  Abs_Diff : Abs  OutDataTypeStr=int32  SaturateOnIntegerOverflow=off
  Const_DiffLe5 : Constant  Value=5  OutDataTypeStr=int32
  Const_One_FailCnt : Constant  OutDataTypeStr=uint32
  Const_One_Hb : Constant  OutDataTypeStr=uint8
  Const_One_HbCnt : Constant  OutDataTypeStr=uint32
  Const_One_IlcCnt : Constant  OutDataTypeStr=uint32
  Const_OpMode1 : Constant  OutDataTypeStr=uint8
  Const_OpMode2 : Constant  Value=2  OutDataTypeStr=uint8
  Const_OpMode3 : Constant  Value=3  OutDataTypeStr=uint8
  Const_OpMode4 : Constant  Value=4  OutDataTypeStr=uint8
  Const_StateFailed : Constant  Value=3  OutDataTypeStr=uint8
  Const_StateHbLost : Constant  Value=2  OutDataTypeStr=uint8
  Const_StateInit : Constant  Value=0  OutDataTypeStr=uint8
  Const_StateOp : Constant  OutDataTypeStr=uint8
  Const_Zero_FailCnt : Constant  Value=0  OutDataTypeStr=uint32
  Const_Zero_HbCnt : Constant  Value=0  OutDataTypeStr=uint32
  Const_Zero_IlcCnt : Constant  Value=0  OutDataTypeStr=uint32
  DTC_HbCntI : DataTypeConversion  OutDataTypeStr=int32  SaturateOnIntegerOverflow=off  RndMeth=Floor
  DTC_IlcCntI : DataTypeConversion  OutDataTypeStr=int32  SaturateOnIntegerOverflow=off  RndMeth=Floor
  DTC_Watch : DataTypeConversion  OutDataTypeStr=uint32  SaturateOnIntegerOverflow=off  RndMeth=Floor
  Delay_FailCnt : UnitDelay  SampleTime=0.01  HasFrameUpgradeWarning=on
  Delay_Hb : UnitDelay  SampleTime=0.01  HasFrameUpgradeWarning=on
  Delay_HbCnt : UnitDelay  SampleTime=0.01  HasFrameUpgradeWarning=on
  Delay_IlcCnt : UnitDelay  SampleTime=0.01  HasFrameUpgradeWarning=on
  Delay_PrevState : UnitDelay  SampleTime=0.01  HasFrameUpgradeWarning=on
  Delay_State : UnitDelay  SampleTime=0.01  HasFrameUpgradeWarning=on
  Logic_CntrInPrgs : Logic  Operator=OR  AllPortsSameDT=off  OutDataTypeStr=boolean
  Logic_CountersActive : Logic  Operator=OR  AllPortsSameDT=off  OutDataTypeStr=boolean
  Logic_EnterFailed : Logic  Inputs=3  AllPortsSameDT=off  OutDataTypeStr=boolean
  Logic_EnterHbLost : Logic  Operator=OR  AllPortsSameDT=off  OutDataTypeStr=boolean
  Logic_EnterOp : Logic  Operator=OR  Inputs=3  AllPortsSameDT=off  OutDataTypeStr=boolean
  Logic_FailCntEn : Logic  AllPortsSameDT=off  OutDataTypeStr=boolean
  Logic_HbCntEn : Logic  AllPortsSameDT=off  OutDataTypeStr=boolean
  Logic_HbLostFromFailed : Logic  AllPortsSameDT=off  OutDataTypeStr=boolean
  Logic_HbLostFromInitOp : Logic  Inputs=3  AllPortsSameDT=off  OutDataTypeStr=boolean
  Logic_IlcCntEn : Logic  AllPortsSameDT=off  OutDataTypeStr=boolean
  Logic_InitActive : Logic  AllPortsSameDT=off  OutDataTypeStr=boolean
  Logic_NotHbOk : Logic  Operator=NOT  Inputs=1  AllPortsSameDT=off  OutDataTypeStr=boolean
  Logic_NotQf : Logic  Operator=NOT  Inputs=1  AllPortsSameDT=off  OutDataTypeStr=boolean
  Logic_OpFromFailed : Logic  AllPortsSameDT=off  OutDataTypeStr=boolean
  Logic_OpFromHbLost : Logic  AllPortsSameDT=off  OutDataTypeStr=boolean
  Logic_OpFromInit : Logic  Inputs=4  AllPortsSameDT=off  OutDataTypeStr=boolean
  Logic_OperModeActive : Logic  Operator=OR  Inputs=4  AllPortsSameDT=off  OutDataTypeStr=boolean
  Logic_StateInitOrOp : Logic  Operator=OR  AllPortsSameDT=off  OutDataTypeStr=boolean
  Relop_DiffLe5 : RelationalOperator  Operator=<=  OutDataTypeStr=boolean  RndMeth=Simplest  InputSameDT=off
  Relop_FailCntWatch : RelationalOperator  OutDataTypeStr=boolean  RndMeth=Simplest  InputSameDT=off
  Relop_HbCntWatch : RelationalOperator  OutDataTypeStr=boolean  RndMeth=Simplest  InputSameDT=off
  Relop_HbOk : RelationalOperator  Operator===  OutDataTypeStr=boolean  RndMeth=Simplest  InputSameDT=off
  Relop_Om{1..4} (4 alike) : RelationalOperator  Operator===  OutDataTypeStr=boolean  RndMeth=Simplest  InputSameDT=off
  Relop_StateFailed : RelationalOperator  Operator===  OutDataTypeStr=boolean  RndMeth=Simplest  InputSameDT=off
  Relop_StateHbLost : RelationalOperator  Operator===  OutDataTypeStr=boolean  RndMeth=Simplest  InputSameDT=off
  Relop_StateInit : RelationalOperator  Operator===  OutDataTypeStr=boolean  RndMeth=Simplest  InputSameDT=off
  Relop_StateOp : RelationalOperator  Operator===  OutDataTypeStr=boolean  RndMeth=Simplest  InputSameDT=off
  Sum_Diff : Sum  Inputs=+-  OutDataTypeStr=int32
  Sum_Expected : Sum  OutDataTypeStr=uint8
  Sum_FailCnt : Sum  OutDataTypeStr=uint32
  Sum_HbCnt : Sum  OutDataTypeStr=uint32
  Sum_IlcCnt : Sum  OutDataTypeStr=uint32
  Sw_FailCnt : Switch  Criteria=u2 ~= 0  OutDataTypeStr=uint32  SaturateOnIntegerOverflow=off  InputSameDT=off
  Sw_HbCnt : Switch  Criteria=u2 ~= 0  OutDataTypeStr=uint32  SaturateOnIntegerOverflow=off  InputSameDT=off
  Sw_IlcCnt : Switch  Criteria=u2 ~= 0  OutDataTypeStr=uint32  SaturateOnIntegerOverflow=off  InputSameDT=off
  Sw_Next1 : Switch  Criteria=u2 ~= 0  OutDataTypeStr=uint8  SaturateOnIntegerOverflow=off  InputSameDT=off
  Sw_Next2 : Switch  Criteria=u2 ~= 0  OutDataTypeStr=uint8  SaturateOnIntegerOverflow=off  InputSameDT=off
  Sw_Next3 : Switch  Criteria=u2 ~= 0  OutDataTypeStr=uint8  SaturateOnIntegerOverflow=off  InputSameDT=off
  Term_LclIlcStatus : Terminator
  cal_u8RmtLaneFailThd : Constant  Description=cal_u8RmtLaneFailThd；故障监控窗口阈值（周期数），对应 P_MLR_RMTLaneFallThd；uint8；单位 cycle；范围 0..255；默认 20  Value=cal_u8RmtLaneFailThd  OutDataTypeStr=uint8
  u8LaneStatus : Outport
  u8PrevLaneStatus : Outport  Port=2
  bLaneStatusCntrInPrgs : Outport  Port=3
  u32HbMonitorCounter : Outport  Port=4
  u32IlcStsMonitorCounter : Outport  Port=5
  u32FailureMonitorCounter : Outport  Port=6
  wires:
  Relop_DiffLe5/1 -> Logic_EnterFailed/2
  Logic_EnterHbLost/1 -> Sw_Next3/2
  Abs_Diff/1 -> Relop_DiffLe5/1
  Logic_HbLostFromInitOp/1 -> Logic_EnterHbLost/1
  Sum_Diff/1 -> Abs_Diff/1
  Relop_HbCntWatch/1 -> Logic_HbLostFromInitOp/2
  Const_DiffLe5/1 -> Relop_DiffLe5/2
  Sum_FailCnt/1 -> Sw_FailCnt/1
  DTC_IlcCntI/1 -> Sum_Diff/2
  Const_One_HbCnt/1 -> Sum_HbCnt/2
  DTC_Watch/1 -> Relop_FailCntWatch/2, Relop_HbCntWatch/2
  Delay_HbCnt/1 -> u32HbMonitorCounter/1, DTC_HbCntI/1, Relop_HbCntWatch/1, Sum_HbCnt/1
  Const_One_FailCnt/1 -> Sum_FailCnt/2
  Sum_IlcCnt/1 -> Sw_IlcCnt/1
  Const_One_IlcCnt/1 -> Sum_IlcCnt/2
  Delay_IlcCnt/1 -> u32IlcStsMonitorCounter/1, DTC_IlcCntI/1, Sum_IlcCnt/1
  Sw_FailCnt/1 -> Delay_FailCnt/1
  Delay_FailCnt/1 -> Relop_FailCntWatch/1, u32FailureMonitorCounter/1, Sum_FailCnt/1
  cal_u8RmtLaneFailThd/1 -> DTC_Watch/1
  Sw_IlcCnt/1 -> Delay_IlcCnt/1
  Const_Zero_FailCnt/1 -> Sw_FailCnt/3
  Const_Zero_IlcCnt/1 -> Sw_IlcCnt/3
  Logic_IlcCntEn/1 -> Sw_IlcCnt/2
  Logic_EnterOp/1 -> Sw_Next1/2
  Sw_Next1/1 -> Delay_State/1
  Const_Zero_HbCnt/1 -> Sw_HbCnt/3
  Logic_OpFromInit/1 -> Logic_EnterOp/1
  Relop_StateFailed/1 -> Logic_HbLostFromFailed/1, Logic_OpFromFailed/1
  Delay_PrevState/1 -> u8PrevLaneStatus/1
  Relop_StateHbLost/1 -> Logic_OpFromHbLost/1
  Relop_StateInit/1 -> Logic_StateInitOrOp/1, Logic_InitActive/1, Logic_OpFromInit/1
  Relop_StateOp/1 -> Logic_StateInitOrOp/2, Logic_CountersActive/2
  Relop_HbOk/1 -> Logic_NotHbOk/1
  Logic_EnterFailed/1 -> Sw_Next2/2
  Relop_Om4/1 -> Logic_OperModeActive/4
  Logic_InitActive/1 -> Logic_CountersActive/1
  Const_OpMode1/1 -> Relop_Om1/2
  Relop_Om1/1 -> Logic_OperModeActive/1
  Delay_State/1 -> Delay_PrevState/1, Relop_StateFailed/1, u8LaneStatus/1, Relop_StateOp/1, Relop_StateHbLost/1, Relop_StateInit/1, Sw_Next3/3
  Sum_Expected/1 -> Relop_HbOk/2
  Logic_HbCntEn/1 -> Sw_HbCnt/2
  Logic_StateInitOrOp/1 -> Logic_HbLostFromInitOp/1, Logic_EnterFailed/1
  bLclIlcStatusQf/1 -> Logic_CntrInPrgs/2, Logic_IlcCntEn/2, Logic_NotQf/1
  Const_OpMode4/1 -> Relop_Om4/2
  Const_OpMode2/1 -> Relop_Om2/2
  Logic_FailCntEn/1 -> Sw_FailCnt/2
  u8OperMode/1 -> Relop_Om4/1, Relop_Om3/1, Relop_Om2/1, Relop_Om1/1
  Sum_HbCnt/1 -> Sw_HbCnt/1
  Const_One_Hb/1 -> Sum_Expected/2
  Const_OpMode3/1 -> Relop_Om3/2
  Logic_NotQf/1 -> Logic_HbLostFromFailed/2, Logic_OpFromInit/3
  Logic_CntrInPrgs/1 -> bLaneStatusCntrInPrgs/1
  Relop_Om2/1 -> Logic_OperModeActive/2
  Logic_OpFromFailed/1 -> Logic_EnterOp/3
  Const_StateHbLost/1 -> Sw_Next3/1, Relop_StateHbLost/2
  DTC_HbCntI/1 -> Sum_Diff/1
  Sw_Next2/1 -> Sw_Next1/3
  u8HeartbeatLostCount/1 -> Delay_Hb/1, Relop_HbOk/1
  Relop_Om3/1 -> Logic_OperModeActive/3
  Logic_CountersActive/1 -> Logic_FailCntEn/1, Logic_IlcCntEn/1, Logic_HbCntEn/1
  Sw_HbCnt/1 -> Delay_HbCnt/1
  Const_StateFailed/1 -> Sw_Next2/1, Relop_StateFailed/2
  Const_StateInit/1 -> Relop_StateInit/2
  Relop_FailCntWatch/1 -> Logic_HbLostFromInitOp/3, Logic_EnterFailed/3
  Delay_Hb/1 -> Sum_Expected/1
  Logic_HbLostFromFailed/1 -> Logic_EnterHbLost/2
  Sw_Next3/1 -> Sw_Next2/3
  Logic_OperModeActive/1 -> Logic_OpFromInit/2, Logic_InitActive/2
  Logic_OpFromHbLost/1 -> Logic_EnterOp/2
  Const_StateOp/1 -> Sw_Next1/1, Relop_StateOp/2
  Logic_NotHbOk/1 -> Logic_HbCntEn/2, Logic_FailCntEn/2, Logic_OpFromFailed/2, Logic_OpFromHbLost/2, Logic_CntrInPrgs/1, Logic_OpFromInit/4
  u8LclIlcStatus/1 -> Term_LclIlcStatus/1

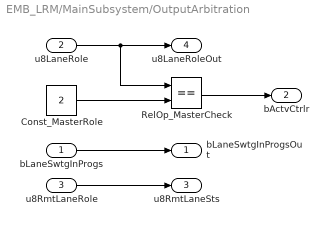
== system EMB_LRM/MainSubsystem/OutputArbitration ==
  bLaneSwtgInProgs : Inport
  u8LaneRole : Inport  Port=2
  u8RmtLaneRole : Inport  Port=3
  Const_MasterRole : Constant  Description=LN_ROLE_MASTER 枚举值 2，用于 bActvCtrlr 判定  Value=2  OutDataTypeStr=uint8
  RelOp_MasterCheck : RelationalOperator  Operator===  OutDataTypeStr=boolean  RndMeth=Simplest  InputSameDT=off
  bLaneSwtgInProgsOut : Outport
  bActvCtrlr : Outport  Port=2
  u8RmtLaneSts : Outport  Port=3
  u8LaneRoleOut : Outport  Port=4
  wires:
  u8RmtLaneRole/1 -> u8RmtLaneSts/1
  RelOp_MasterCheck/1 -> bActvCtrlr/1
  bLaneSwtgInProgs/1 -> bLaneSwtgInProgsOut/1
  Const_MasterRole/1 -> RelOp_MasterCheck/2
  u8LaneRole/1 -> RelOp_MasterCheck/1, u8LaneRoleOut/1

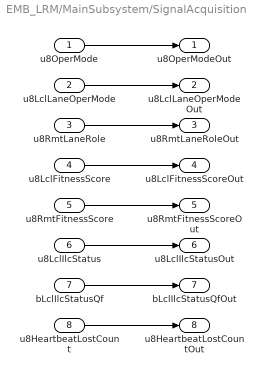
== system EMB_LRM/MainSubsystem/SignalAcquisition ==
  u8OperMode : Inport
  u8LclLaneOperMode : Inport  Port=2
  u8RmtLaneRole : Inport  Port=3
  u8LclFitnessScore : Inport  Port=4
  u8RmtFitnessScore : Inport  Port=5
  u8LclIlcStatus : Inport  Port=6
  bLclIlcStatusQf : Inport  Port=7
  u8HeartbeatLostCount : Inport  Port=8
  u8OperModeOut : Outport
  u8LclLaneOperModeOut : Outport  Port=2
  u8RmtLaneRoleOut : Outport  Port=3
  u8LclFitnessScoreOut : Outport  Port=4
  u8RmtFitnessScoreOut : Outport  Port=5
  u8LclIlcStatusOut : Outport  Port=6
  bLclIlcStatusQfOut : Outport  Port=7
  u8HeartbeatLostCountOut : Outport  Port=8
  wires:
  u8HeartbeatLostCount/1 -> u8HeartbeatLostCountOut/1
  u8LclLaneOperMode/1 -> u8LclLaneOperModeOut/1
  u8LclFitnessScore/1 -> u8LclFitnessScoreOut/1
  u8RmtLaneRole/1 -> u8RmtLaneRoleOut/1
  bLclIlcStatusQf/1 -> bLclIlcStatusQfOut/1
  u8OperMode/1 -> u8OperModeOut/1
  u8LclIlcStatus/1 -> u8LclIlcStatusOut/1
  u8RmtFitnessScore/1 -> u8RmtFitnessScoreOut/1

== stateflow chart EMB_LRM/MainSubsystem/LRM_MLR_ManageLaneRole/MLR_STM ==
  state INIT
    en: u8LaneRole = 1;
  state MASTER
    en: u8LaneRole = 2;
  state FALLBACK
    en: u8LaneRole = 3;
  state SUPPORT
    en: u8LaneRole = 4;
  state DISABLED
    en: u8LaneRole = 5;
  state SHUTTING_DOWN
    en: u8LaneRole = 6;
  (default) -> INIT
  DISABLED -> DISABLED [order 2] : [bLclDisabled]
  SHUTTING_DOWN -> SHUTTING_DOWN [order 2] : [bOperShutdown]
  MASTER -> FALLBACK [order 4] : [bMasterToFallbackImm]
  INIT -> MASTER [order 3] : [bExitInitMaster]
  INIT -> FALLBACK [order 4] : [bExitInitFallback]
  FALLBACK -> MASTER [order 3] : [bFbToMasterImm]
  FALLBACK -> MASTER [order 4] : [bFbToMasterTakeover]
  MASTER -> FALLBACK [order 5] : [bMasterToFallbackCnt]
  FALLBACK -> SUPPORT [order 5] : [bFbToSupport]
  FALLBACK -> SUPPORT [order 6] : [bFbToSupportFail]
  SHUTTING_DOWN -> INIT [order 3] : [bNotOperShutdown]
  MASTER -> SUPPORT [order 3] : [bMasterToSupport]
  FALLBACK -> DISABLED [order 2] : [bLclDisabled]
  INIT -> SHUTTING_DOWN [order 1] : [bOperShutdown]
  INIT -> DISABLED [order 2] : [bLclDisabled]
  SUPPORT -> MASTER [order 3] : [bFbToMasterImm]
  SUPPORT -> MASTER [order 4] : [bSpToMasterTakeover]
  SUPPORT -> FALLBACK [order 5] : [bSpToFallback]
  MASTER -> DISABLED [order 2] : [bLclDisabled]
  MASTER -> SHUTTING_DOWN [order 1] : [bOperShutdown]
  FALLBACK -> SHUTTING_DOWN [order 1] : [bOperShutdown]
  SUPPORT -> SHUTTING_DOWN [order 1] : [bOperShutdown]
  DISABLED -> SHUTTING_DOWN [order 1] : [bOperShutdown]
  SUPPORT -> DISABLED [order 2] : [bLclDisabled]
  SHUTTING_DOWN -> DISABLED [order 1] : [bLclDisabled]
  data: bOperShutdown input boolean; bLclDisabled input boolean; bLclGtRmt input boolean; bLclLtRmt input boolean; bRmtMaster input boolean; bRmtFallback input boolean; bRmtDisabled input boolean; bRmtShutdown input boolean; bRmtUnknown input boolean; bIlcFailed input boolean; bLaneStsFailed input boolean; bRmtScoreValid input boolean; bNotOperShutdown input boolean; bNotRmtMaster input boolean; bNotIlcFailed input boolean; bExitInitMaster input boolean; bExitInitFallback input boolean; bMasterToSupport input boolean; bMasterToFallbackImm input boolean; bMasterToFallbackCnt input boolean; bFbToMasterImm input boolean; bFbToMasterTakeover input boolean; bFbToSupport input boolean; bFbToSupportFail input boolean; bSpToMasterTakeover input boolean; bSpToFallback input boolean; u8LaneRole output uint8 =1
